simulink model "hybrid_force_pos_controller"  (R2021b)
settings: Solver=VariableStepAuto  StartTime=0.0  StopTime=10.0  RelTol=1e-3
values from neighbouring files (symbols this model uses):
  constraint_matrix = diag([0 0 1 0 0 0])    [lfd_force_estimation.m]    (also in lfd_real_data.m)
  ik_weights = [1 1 1 1 1 1]    [lfd_force_estimation.m]    (also in lfd_real_data.m; test_inverse_kinematics.m)
  invMd = inv(Md)    [lfd_force_estimation.m]    (also in lfd_real_data.m)
  K = 5    [lfd_demo.m]    (also in lfd_force_estimation.m = [0 0 0 0 0 0; lfd_real_data.m = [0 0 0 0 0 0; lfd_ur_robot.m)
  kd = [5 0 0 0 0 0 ... (first row only)    [lfd_force_estimation.m]    (also in lfd_real_data.m)
  kif = [0.001 0 0 0 0 0 ... (first row only)    [lfd_force_estimation.m]    (also in lfd_real_data.m = [0.01 0 0 0 0 0)
  kp = [10 0 0 0 0 0 ... (first row only)    [lfd_force_estimation.m]    (also in lfd_real_data.m)
  kpf = [0.1 0 0 0 0 0 ... (first row only)    [lfd_force_estimation.m]    (also in lfd_real_data.m)
undefined symbols (not defined in the file or in its folder): config
libraries: robotmaniplib x4, robotcorelib x2, dspmtrx3 x2
settings Model: Creator=peter  LastModifiedBy=peter

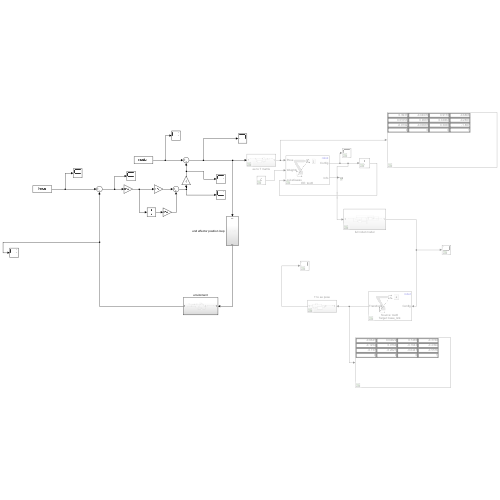
[thumbnail: Simulink's stored preview of the top-level diagram]
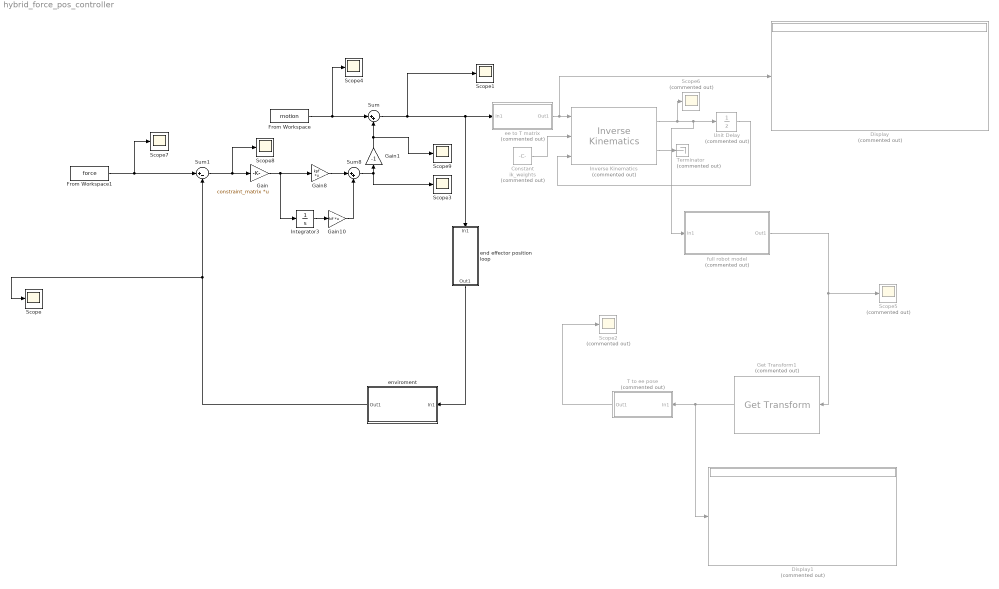
== system hybrid_force_pos_controller ==
  Constant : Constant  Commented=on  Value=ik_weights
  Display : Display  Commented=on
  Display1 : Display  Commented=on
  From Workspace : FromWorkspace  VariableName=motion
  From Workspace1 : FromWorkspace  VariableName=force
  Gain : Gain  Gain=constraint_matrix  Multiplication=Matrix(K*u)
  Gain1 : Gain  Gain=-1
  Gain10 : Gain  Gain=kif  Multiplication=Matrix(K*u)
  Gain8 : Gain  Gain=kpf  Multiplication=Matrix(K*u)
  Get Transform1 : robotmaniplib/Get Transform  Commented=on  RigidBodyTree=robot  SourceBody=tool0  TargetBody=base_link  SimulateUsing=Interpreted execution
  Integrator3 : Integrator
  Inverse Kinematics : robotmaniplib/Inverse Kinematics  Commented=on  RigidBodyTree=robot  EndEffector=tool0  ShowInfo=on  SolverName=BFGS Gradient Projection  EnforceJointLimits=on  MaxIterations=1500  MaxTime=10  GradientTolerance=1e-7  SolutionTolerance=1e-6  StepTolerance=1e-14  ErrorChangeTolerance=1e-12  UseErrorDamping=on  DampingBias=0.0025  SimulateUsing=Interpreted execution
  Scope{,1,3..4,7..9} (7 alike) : Scope
  Scope2 : Scope  Commented=on
  Scope5 : Scope  Commented=on
  Scope6 : Scope  Commented=on
  Sum : Sum  Inputs=|++
  Sum1 : Sum  Inputs=|+-
  Sum8 : Sum  Inputs=|++
  T to ee pose : Subsystem  Commented=on
  Terminator : Terminator  Commented=on
  Unit Delay : UnitDelay  Commented=on  SampleTime=-1  HasFrameUpgradeWarning=on
  ee to T matrix : Subsystem  Commented=on
  end effector position loop : Subsystem
  enviroment : Subsystem
  full robot model : Subsystem  Commented=on
  wires:
  From Workspace/1 -> Scope4/1, Sum/1
  Sum1/1 -> Scope8/1, Gain/1
  Gain8/1 -> Sum8/1
  Gain10/1 -> Sum8/2
  Integrator3/1 -> Gain10/1
  Gain/1 -> Integrator3/1, Gain8/1
  Sum8/1 -> Scope3/1, Gain1/1
  Sum/1 -> Scope1/1, ee to T matrix/1(In1), end effector position loop/1(In1)
  Get Transform1/1 -> Display1/1, T to ee pose/1(In1)
  From Workspace1/1 -> Scope7/1, Sum1/1
  ee to T matrix/1(Out1) -> Display/1, Inverse Kinematics/1
  Constant/1 -> Inverse Kinematics/2
  Unit Delay/1 -> Inverse Kinematics/3
  Inverse Kinematics/2 -> Terminator/1
  enviroment/1(Out1) -> Sum1/2, Scope/1
  T to ee pose/1(Out1) -> Scope2/1
  Inverse Kinematics/1 -> full robot model/1(In1), Unit Delay/1, Scope6/1
  full robot model/1(Out1) -> Scope5/1, Get Transform1/1
  Gain1/1 -> Scope9/1, Sum/2
  end effector position loop/1(Out1) -> enviroment/1(In1)

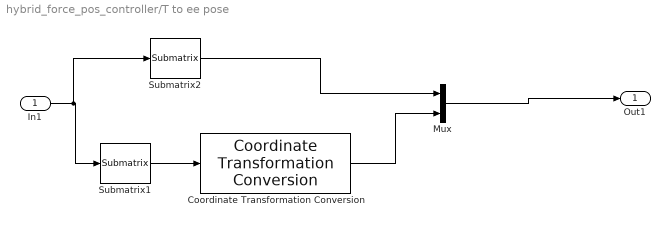
== system hybrid_force_pos_controller/T to ee pose ==
  In1 : Inport
  Coordinate Transformation Conversion : robotcorelib/Coordinate Transformation Conversion  InputRepresentation=Rotation Matrix  InputEulerSequence=ZYX  ShowTrVecInputPort=on  OutputRepresentation=Euler Angles  OutputEulerSequence=ZYX  ShowTrVecOutputPort=on  SimulateUsing=Interpreted execution
      settings: SourceProductBaseCode=NV,RO,RR,UV
  Mux : Mux  Inputs=2
  Submatrix1 : dspmtrx3/Submatrix  RowSpan=Range of rows  RowStartMode=First  RowStartIndex=4  RowEndMode=Index  RowEndIndex=3  ColSpan=Range of columns  ColStartMode=First  ColStartIndex=4  ColEndMode=Index  ColEndIndex=3
  Submatrix2 : dspmtrx3/Submatrix  RowSpan=Range of rows  RowStartMode=First  RowStartIndex=4  RowEndMode=Index  RowEndIndex=3  ColSpan=Range of columns  ColStartMode=Index  ColStartIndex=4  ColEndMode=Index  ColEndIndex=4
  Out1 : Outport
  wires:
  In1/1 -> Submatrix2/1, Submatrix1/1
  Submatrix1/1 -> Coordinate Transformation Conversion/1
  Coordinate Transformation Conversion/1 -> Mux/2
  Mux/1 -> Out1/1
  Submatrix2/1 -> Mux/1

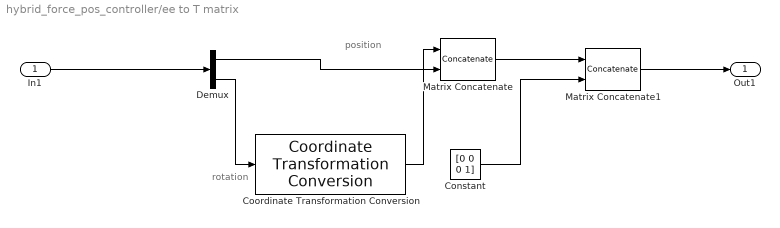
== system hybrid_force_pos_controller/ee to T matrix ==
  note: position
  note: rotation
  In1 : Inport
  Constant : Constant  Value=[0 0 0 1]  VectorParams1D=off
  Coordinate Transformation Conversion : robotcorelib/Coordinate Transformation Conversion  InputRepresentation=Euler Angles  InputEulerSequence=ZYX  ShowTrVecInputPort=on  OutputRepresentation=Rotation Matrix  OutputEulerSequence=ZYX  ShowTrVecOutputPort=on  SimulateUsing=Interpreted execution
      settings: SourceProductBaseCode=NV,RO,RR,UV
  Demux : Demux  Outputs=2
  Matrix Concatenate : Concatenate  Mode=Multidimensional array  ConcatenateDimension=2
  Matrix Concatenate1 : Concatenate  Mode=Multidimensional array
  Out1 : Outport
  wires:
  Demux/2 -> Coordinate Transformation Conversion/1
  Coordinate Transformation Conversion/1 -> Matrix Concatenate/1
  Demux/1 -> Matrix Concatenate/2
  In1/1 -> Demux/1
  Matrix Concatenate/1 -> Matrix Concatenate1/1
  Constant/1 -> Matrix Concatenate1/2
  Matrix Concatenate1/1 -> Out1/1

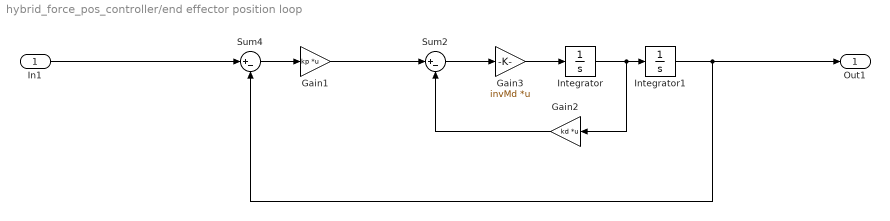
== system hybrid_force_pos_controller/end effector position loop ==
  In1 : Inport
  Gain1 : Gain  Gain=kp  Multiplication=Matrix(K*u)
  Gain2 : Gain  Gain=kd  Multiplication=Matrix(K*u)
  Gain3 : Gain  Gain=invMd  Multiplication=Matrix(K*u)
  Integrator : Integrator
  Integrator1 : Integrator
  Sum2 : Sum  Inputs=|+-
  Sum4 : Sum  Inputs=|+-
  Out1 : Outport
  wires:
  Sum4/1 -> Gain1/1
  Gain1/1 -> Sum2/1
  Gain3/1 -> Integrator/1
  Sum2/1 -> Gain3/1
  Gain2/1 -> Sum2/2
  Integrator/1 -> Gain2/1, Integrator1/1
  Integrator1/1 -> Sum4/2, Out1/1
  In1/1 -> Sum4/1

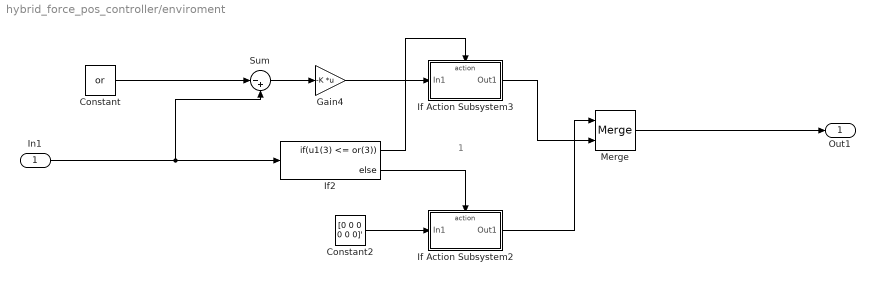
== system hybrid_force_pos_controller/enviroment ==
  note: 1
  In1 : Inport
  Constant : Constant  Value=or
  Constant2 : Constant  Value=[0 0 0 0 0 0]'  VectorParams1D=off
  Gain4 : Gain  Gain=-K  Multiplication=Matrix(K*u)
  If Action Subsystem2 : Subsystem  TreatAsAtomicUnit=on
  If Action Subsystem3 : Subsystem  TreatAsAtomicUnit=on
  If2 : If  IfExpression=u1(3) <= or(3)
  Merge : Merge
  Sum : Sum  Inputs=|-+
  Out1 : Outport
  wires:
  If2/2 -> If Action Subsystem2/Action
  Gain4/1 -> If Action Subsystem3/1(In1)
  Constant2/1 -> If Action Subsystem2/1(In1)
  If Action Subsystem3/1(Out1) -> Merge/2
  If2/1 -> If Action Subsystem3/Action
  If Action Subsystem2/1(Out1) -> Merge/1
  Merge/1 -> Out1/1
  Sum/1 -> Gain4/1
  Constant/1 -> Sum/1
  In1/1 -> Sum/2, If2/1

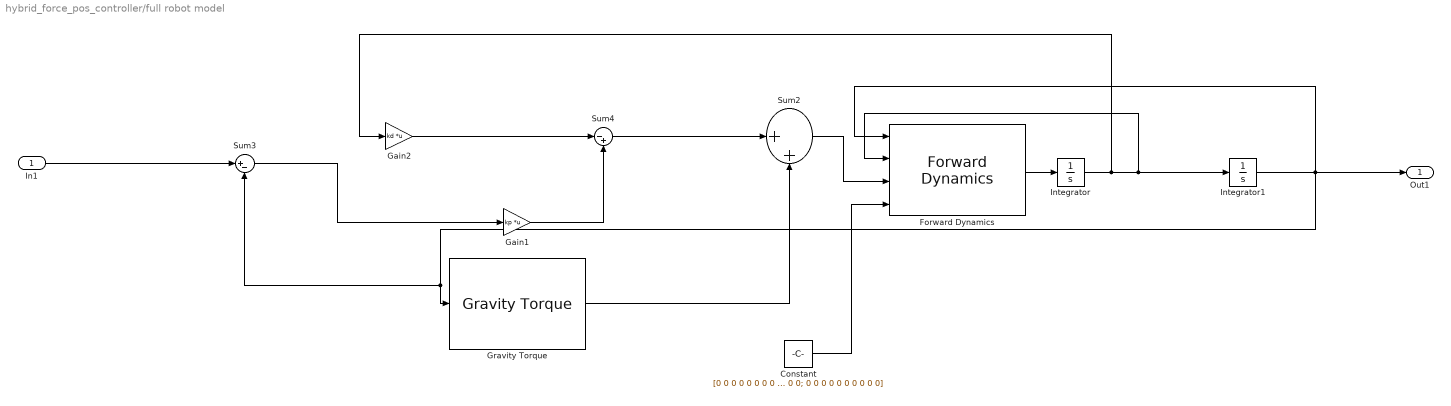
== system hybrid_force_pos_controller/full robot model ==
  In1 : Inport
  Constant : Constant  Value=[0 0 0 0 0 0 0 0 0 0; 0 0 0 0 0 0 0 0 0 0; 0 0 0 0 0 0 0 0 0 0; 0 0 0 0 0 0 0 0 0 0; 0 0 0 0 0 0 0 0 0 0; 0 0 0 0 0 0 0 0 0 0]
  Forward Dynamics : robotmaniplib/Forward Dynamics  RigidBodyTree=robot  SimulateUsing=Interpreted execution
  Gain1 : Gain  Gain=kp  Multiplication=Matrix(K*u)
  Gain2 : Gain  Gain=kd  Multiplication=Matrix(K*u)
  Gravity Torque : robotmaniplib/Gravity Torque  RigidBodyTree=robot  SimulateUsing=Interpreted execution
  Integrator : Integrator
  Integrator1 : Integrator  InitialCondition=config
  Sum2 : Sum  Inputs=|++
  Sum3 : Sum  Inputs=|+-
  Sum4 : Sum  Inputs=|-+
  Out1 : Outport
  wires:
  In1/1 -> Sum3/1
  Sum3/1 -> Gain1/1
  Gravity Torque/1 -> Sum2/2
  Gain1/1 -> Sum4/2
  Sum2/1 -> Forward Dynamics/3
  Sum4/1 -> Sum2/1
  Integrator/1 -> Gain2/1, Forward Dynamics/2, Integrator1/1
  Gain2/1 -> Sum4/1
  Forward Dynamics/1 -> Integrator/1
  Constant/1 -> Forward Dynamics/4
  Integrator1/1 -> Forward Dynamics/1, Sum3/2, Gravity Torque/1, Out1/1

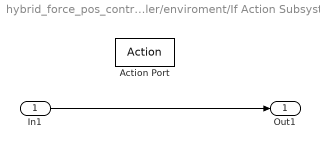
== system hybrid_force_pos_controller/enviroment/If Action Subsystem2 ==
  In1 : Inport
  Action Port : ActionPort  ActionPortLabel=else
  Out1 : Outport
  wires:
  In1/1 -> Out1/1

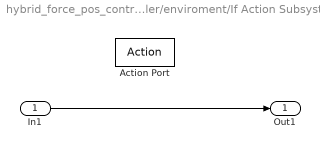
== system hybrid_force_pos_controller/enviroment/If Action Subsystem3 ==
  In1 : Inport
  Action Port : ActionPort  ActionPortLabel=if(u1(3) <= or(3))
  Out1 : Outport
  wires:
  In1/1 -> Out1/1
